simulink model "desorption_03c_sim_cl"  (R2017b)
settings: Solver=ode23s  StartTime=0.0  StopTime=tEndSimul  MaxStep=0.1  RelTol=1e-4
values from neighbouring files (symbols this model uses):
  b_motor = 1e-3    (= 0.001)    [desorption_03c_cl.m]
  c = conversion_factors()    [desorption_03c_cl.m]
  compr_water_epsilon = 0.8    [desorption_03c_cl.m]
  compr_water_flow_L_min = 10    [desorption_03c_cl.m]
  compr_water_Tin_C = Tamb_C    (= 25)    [desorption_03c_cl.m]
  fluid = nh3_v4    [desorption_03c_cl.m]
  h_liq_wall = 50    [desorption_03c_cl.m]
  h_reactor_air = h_desorp    (= 200)    [desorption_03c_cl.m]
  h_reservoir_inner_liq = 50    [desorption_03c_cl.m]
  h_reservoir_inner_vap = 10    [desorption_03c_cl.m]
  h_reservoir_outer = 10    [desorption_03c_cl.m]
  h_vap_wall = 1e4    (= 10000)    [desorption_03c_cl.m]
  h_wall_water = 200    [desorption_03c_cl.m]
  J_motor = 0.1    [desorption_03c_cl.m]
  L_min_water = L_min_water_condenser    (= 20)    [desorption_03c_cl.m]
  La_motor = 2.31e-3    (= 0.00231)    [desorption_03c_cl.m]
  motor_start_time_sec = 100 * c.min_to_sec    [desorption_03c_cl.m]
  PID_I_Tdisch = 0.01    [desorption_03c_cl.m]
  PID_P_Tdisch = 5    [desorption_03c_cl.m]
  Ra_motor = 2    [desorption_03c_cl.m]
  reservoir_L = 0.4 * Ngalettes * 46.5 * c.mm_to_m    [desorption_03c_cl.m]
  rpm_init = 0    [desorption_03c_cl.m]
  rpm_max = dVswept_rmp * 2    (= 2900)    [desorption_03c_cl.m]
  T1 = motor_start_time_sec+0    [desorption_03c_cl.m]
  Tamb_C = 25    [desorption_03c_cl.m]
  Tdesorp_source_C = Tdesorp_C    (= 25)    [desorption_03c_cl.m]
  Tdisch_ref_C = Tdisch    (= 180)    [desorption_03c_cl.m]
  Twater_in_C = 25    [desorption_03c_cl.m]
  Xend = Xinit - 0.9    (= 0.09)    [desorption_03c_cl.m]
undefined symbols (not defined in the file or in its folder): PID_D_Tdisch
libraries: thermochemical x41, simulink_extras x4, simulink x2
settings Model: Creator=ferru  LastModifiedBy=fferrucc
settings SolverCC: ZeroCrossAlgorithm=Adaptive

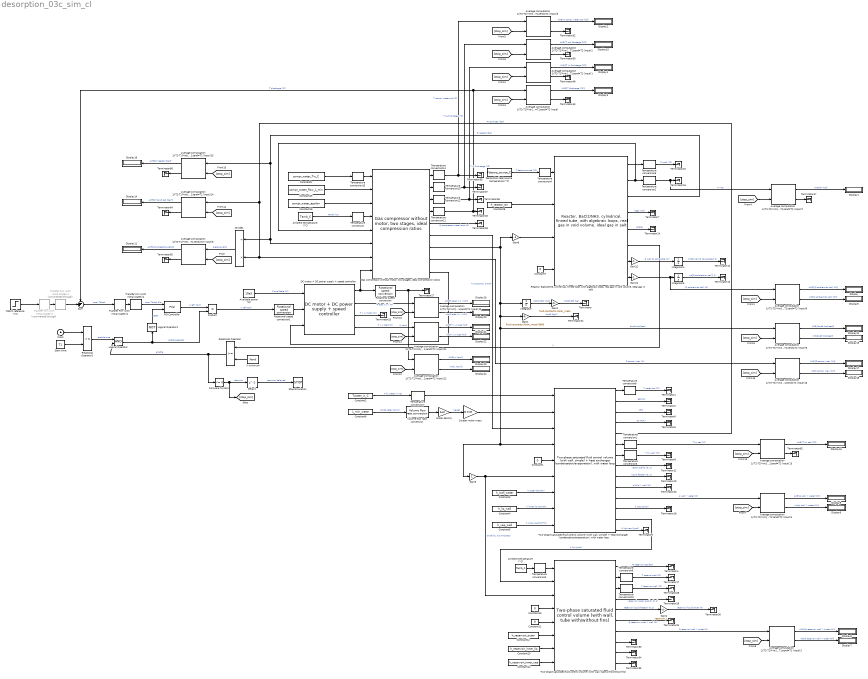
== system desorption_03c_sim_cl ==
  1/water molar mass : Gain  Gain=55.5085
  Ambient temperature (°C) : Constant  Value=Tamb_C
  "Ambient temperature (°C) " : Constant  Value=Tamb_C
  Available power (W) : Constant  Value=10e3
  Average computation 1/(T2-T1)*int{x}|t0=T1,tend=T2 (input){,1..16} (17 alike) : thermochemical/Utils/Average computation 1//(T2-T1)*int{x}|t0=T1,tend=T2 (input)  T1=T1
      settings: SourceProductName=@ Thermochemical
  Clock : Clock
  Compare To Zero : simulink/Logic and Bit Operations/Compare To Zero  relop=<=  OutDataTypeStr=boolean
  Constant{1,7,10..11} (4 alike) : Constant  Value=0
  Constant12 : Constant  Value=h_reservoir_outer
  Constant13 : Constant  Value=h_reservoir_inner_liq
  Constant14 : Constant  Value=h_reservoir_inner_vap
  Constant15 : Constant  Value=compr_water_flow_L_min
  Constant16 : Constant  Value=compr_water_epsilon
  Constant2 : Constant  Value=Twater_in_C
  Constant3 : Constant  Value=h_wall_water
  Constant4 : Constant  Value=h_liq_wall
  Constant5 : Constant  Value=h_vap_wall
  Constant6 : Constant  Value=L_min_water
  Constant8 : Constant  Value=h_reactor_air
  Constant9 : Constant  Value=compr_water_Tin_C
  DC motor + DC power supply + speed controller : thermochemical/Motors/DC motor + DC power supply +  speed controller  L=La_motor  R=Ra_motor  J=J_motor  b=b_motor  Km=Km_motor  w_init_motor=rpm_init*c.rpm_to_rad_sec  PID_P=PID_P_motor  PID_I=PID_I_motor  PID_D=PID_D_motor  V_max=Vmax_motor
      settings: SourceProductName=@ Thermochemical
  Delay1 : Delay  DelayLength=1
  Desorption heat source temperature (°C) : Constant  Value=Tdesorp_source_C
  Display{,1..24} (25 alike) : Display
  Divide1 : Product  Inputs=/*
  Gain1 : Gain  Gain=fluid.constants.Molar_mass*3600
  Gain11 : Gain  Gain=-1
  Gain12 : Gain  Gain=-1
  Gain2 : Gain  Gain=fluid.constants.Molar_mass
  Gain3 : Gain
  Gain4 : Gain  Gain=reservoir_L
  Gain6 : Gain  Gain=-1
  "Gas compressor without motor, two stages, ideal compression ratios" : thermochemical/Compression/Gas compressor without motor, two stages, ideal compression ratios  fluid=fluid  eta_IS=0.7  CL=0.03  eta_mech=0.9  dVswept_m3_h=6  dVswept_rmp=1500
      settings: SourceProductName=@ Thermochemical
  Integrator : Integrator
  Integrator4 : Integrator
  Integrator5 : Integrator
  Logical Operator : Logic  AllPortsSameDT=off  OutDataTypeStr=boolean
  Logical Operator1 : Logic  Operator=NOT  AllPortsSameDT=off  OutDataTypeStr=boolean
  PID Controller : simulink/Continuous/PID Controller  Controller=PI  TimeDomain=Continuous-time  SampleTime=-1  IntegratorMethod=Forward Euler  FilterMethod=Forward Euler  Form=Ideal  UseFilter=on  ControllerParametersSource=internal  P=PID_P_Tdisch  I=PID_I_Tdisch  D=PID_D_Tdisch  N=100  InitialConditionSource=internal  InitialConditionForIntegrator=0  InitialConditionForFilter=0  ExternalReset=level  LimitOutput=on  UpperSaturationLimit=rpm_max  LowerSaturationLimit=0  LinearizeAsGain=off  AntiWindupMode=clamping  Kb=1  TrackingMode=off  Kt=1  PParamMin=[]  PParamMax=[]  IParamMin=[]  IParamMax=[]  DParamMin=[]  DParamMax=[]  NParamMin=[]  NParamMax=[]  KbParamMin=[]  KbParamMax=[]  KtParamMin=[]  KtParamMax=[]  POutMin=[]  POutMax=[]  IOutMin=[]  IOutMax=[]  DOutMin=[]  DOutMax=[]  NOutMin=[]  NOutMax=[]  KbOutMin=[]  KbOutMax=[]  KtOutMin=[]  KtOutMax=[]  IntegratorOutMin=[]  IntegratorOutMax=[]  FilterOutMin=[]  FilterOutMax=[]  SumOutMin=[]  SumOutMax=[]  SumI1OutMin=[]  SumI1OutMax=[]  SumI2OutMin=[]  SumI2OutMax=[]  SumI3OutMin=[]  SumI3OutMax=[]  SumDOutMin=[]  SumDOutMax=[]  SaturationOutMin=[]  SaturationOutMax=[]  IntegratorContinuousStateAttributes=''  IntegratorStateMustResolveToSignalObject=off  IntegratorRTWStateStorageClass=Auto  FilterContinuousStateAttributes=''  FilterStateMustResolveToSignalObject=off  FilterRTWStateStorageClass=Auto  DifferentiatorICPrevScaledInput=0  DifferentiatorOutMin=[]  DifferentiatorOutMax=[]  InitialConditionSetting=State (most efficient)  FilterDiffOutCoefMin=[]  FilterDiffOutCoefMax=[]  SumDenOutMin=[]  SumDenOutMax=[]  SumNumOutMin=[]  SumNumOutMax=[]  ReciprocalOutMin=[]  ReciprocalOutMax=[]  DivideOutMin=[]  DivideOutMax=[]  TunerSelectOption=Transfer Function Based (PID Tuner App)
  Product : Product
  "Reactor, BaCl2/NH3, cylindrical, finned tube, with algebraic loops, real gas in void volume, ideal gas in salt" : thermochemical/Reactors/Reactor, BaCl2//NH3, with algebraic loops, real gas in void volume, ideal gas in salt/Reactor, BaCl2//NH3, cylindrical, finned tube, with algebraic loops, real gas in void volume, ideal gas in salt
      link override "Reactor, BaCl2//NH3, cylindrical, no walls, with algebraic loops, real gas in void volume, ideal gas in salt": tao_salt=param.tao_salt  rho_composite=param.rho_composite  K_cin=K_cin  fluid=fluid  Lr=param.Lr  Lr_total=param.Lr_total  Dr=param.D  Ddiff=param.Ddiff  Tr_init=param.Tr_init  X_init=param.X_init
      link override "Wall, tube with//without fins": L_m=param.Lr_total  OD_mm=OD_mm  e_mm=thickness_mm  Tinit=Treactor_wall_init  height_fin_mm=0  thickness_fin_mm=0  pitch_fin_mm=0  material_fin=Aluminum 1100  cp_fin=905.9  rho_fin=2658  lambda_fin=211.8
      settings: SourceProductName=@ Thermochemical
  Relational Operator : RelationalOperator  OutDataTypeStr=boolean  RndMeth=Simplest
  Relational Operator1 : RelationalOperator  OutDataTypeStr=boolean  RndMeth=Simplest
  Rotational speed conversion : thermochemical/Conversions/Rotational speed conversion  sel=rad/sec --> rpm
      settings: SourceProductName=@ Thermochemical
  Rotational speed conversion1 : thermochemical/Conversions/Rotational speed conversion  sel=rpm --> rad/sec
      settings: SourceProductName=@ Thermochemical
  Start time : Constant  Value=T1
  Stop Simulation : Stop
  Sum : Sum  Inputs=-+|
  Tdisch reference (°C) : Step  Time=motor_start_time_sec  Before=Tamb_C  After=Tdisch_ref_C  SampleTime=0
  Temperature conversion{,4..5,7,15} (5 alike) : thermochemical/Conversions/Temperature conversion  sel=°C --> K
      settings: SourceProductName=@ Thermochemical
  Temperature conversion{1..3,6,8..14} (11 alike) : thermochemical/Conversions/Temperature conversion  sel=K --> °C
      settings: SourceProductName=@ Thermochemical
  Terminator{,1..2,4..18,20,22,25..31,33..39,43,47..48,50,52,55,62,64,66} (43 alike) : Terminator
  Transfer Fcn (with initial states)1 : simulink_extras/Additional Linear/Transfer Fcn (with initial states)  N=[1]  D="[5  1]"  X0=0
  Transfer Fcn (with initial states)2 : simulink_extras/Additional Linear/Transfer Fcn (with initial states)  N=[1]  D="[5  1]"  X0=0
  Transfer Fcn (with initial states)3 : simulink_extras/Additional Linear/Transfer Fcn (with initial states)  Commented=through  N=[1]  D="[5  1]"  X0=Tamb_C
  Transfer Fcn (with initial states)4 : simulink_extras/Additional Linear/Transfer Fcn (with initial states)  Commented=through  N=[1]  D="[5  1]"  X0=Tamb_C
  "Two-phase saturated fluid control volume (with wall, tube with/without fins)" : thermochemical/Control volumes/Two-phase saturated fluid control volume (with wall, tube with//without fins)
      link override Two-phase saturated fluid control volume (without walls): N_init=reservoir_Ninit  T_init=reservoir_Tinit  V=reservoir_V
      link override "Wall, tube with//without fins": L_m=reservoir_L  OD_mm=reservoir_OD_mm  e_mm=reservoir_thickness_mm  material_tube=Stainless steel AISI316  cp_tube=490.8  rho_tube=8023
      settings: SourceProductName=@ Thermochemical
  "Two-phase saturated fluid control volume (with wall, simple) + heat exchanger (condensation/evaporation), with water loop" : thermochemical/Control volumes/Two-phase saturated fluid control volume (with wall, simple) + heat exchanger (condensation//evaporation), with water loop
      link override "Two-phase saturated fluid control volume (with wall, simple)/Two-phase saturated fluid control volume (without walls)": N_init=Nhx_init  T_init=Thx_init  V=Vhx
      link override "Two-phase saturated fluid control volume (with wall, simple)/Wall, simple, h as inputs": material=Stainless steel AISI316  cp=490.8  rho=8023  s=Shx_m2  e_mm=thickness_hx_mm  mass=2.2529
      settings: SourceProductName=@ Thermochemical
  Volume flow rate conversion : thermochemical/Conversions/Volume flow rate conversion  sel=L/min --> m3/sec
      settings: SourceProductName=@ Thermochemical
  Water density : Gain  Gain=1e3
  X minimum : Constant  Value=Xend
  wires:
  Integrator/1 -> Gain2/1  "int{dn/dt} (mol)"
  Temperature conversion2/1 -> "Average computation 1/(T2-T1)*int{x}|t0=T1,tend=T2 (input)7"/1, Terminator16/1  "Tr (°C)"
  Temperature conversion6/1 -> Terminator15/1  "Tr,wall (°C)"
  "Reactor, BaCl2/NH3, cylindrical, finned tube, with algebraic loops, real gas in void volume, ideal gas in salt"/4 -> Terminator7/1  "hgas void"
  "Reactor, BaCl2/NH3, cylindrical, finned tube, with algebraic loops, real gas in void volume, ideal gas in salt"/5 -> Terminator14/1  "phase"
  "Reactor, BaCl2/NH3, cylindrical, finned tube, with algebraic loops, real gas in void volume, ideal gas in salt"/2 -> "Gas compressor without motor, two stages, ideal compression ratios"/5, Temperature conversion2/1
  "Reactor, BaCl2/NH3, cylindrical, finned tube, with algebraic loops, real gas in void volume, ideal gas in salt"/6 -> Relational Operator/1  "X"
  "Reactor, BaCl2/NH3, cylindrical, finned tube, with algebraic loops, real gas in void volume, ideal gas in salt"/3 -> "Average computation 1/(T2-T1)*int{x}|t0=T1,tend=T2 (input)15"/1, Divide1/1, "Gas compressor without motor, two stages, ideal compression ratios"/6  "Pr reactor (bar)"
  "Reactor, BaCl2/NH3, cylindrical, finned tube, with algebraic loops, real gas in void volume, ideal gas in salt"/1 -> Temperature conversion6/1
  Gain11/1 -> "Average computation 1/(T2-T1)*int{x}|t0=T1,tend=T2 (input)6"/1, Integrator5/1  "Q ambient to wall (W)"
  "Reactor, BaCl2/NH3, cylindrical, finned tube, with algebraic loops, real gas in void volume, ideal gas in salt"/8 -> Gain11/1
  Integrator4/1 -> Terminator12/1  "int{Q wall to composite} (J)"
  Gain12/1 -> Integrator4/1  "Q wall to composite (W)"
  Integrator5/1 -> Terminator13/1  "int{Q ambient to wall} (J)"
  "Reactor, BaCl2/NH3, cylindrical, finned tube, with algebraic loops, real gas in void volume, ideal gas in salt"/7 -> Gain12/1
  "Two-phase saturated fluid control volume (with wall, simple) + heat exchanger (condensation/evaporation), with water loop"/10 -> Terminator20/1  "q fluid > wall (W)"
  "Two-phase saturated fluid control volume (with wall, simple) + heat exchanger (condensation/evaporation), with water loop"/9 -> Terminator10/1  "liquid fraction (0..1)"
  Water density/1 -> 1/water molar mass/1  "kg/sec"
  Temperature conversion3/1 -> Terminator8/1  "T hx,wall (°C)"
  "Two-phase saturated fluid control volume (with wall, simple) + heat exchanger (condensation/evaporation), with water loop"/11 -> "Average computation 1/(T2-T1)*int{x}|t0=T1,tend=T2 (input)4"/1  "q wall > water (W)"
  Constant2/1 -> Temperature conversion7/1  "T hx,water in (°C)"
  "Two-phase saturated fluid control volume (with wall, simple) + heat exchanger (condensation/evaporation), with water loop"/2 -> Terminator2/1  "epsilon"
  "Two-phase saturated fluid control volume (with wall, simple) + heat exchanger (condensation/evaporation), with water loop"/4 -> Terminator5/1  "UA (W/K)"
  "Two-phase saturated fluid control volume (with wall, simple) + heat exchanger (condensation/evaporation), with water loop"/12 -> Terminator18/1  "h vap (J/mol)"
  "Two-phase saturated fluid control volume (with wall, simple) + heat exchanger (condensation/evaporation), with water loop"/1 -> Temperature conversion8/1
  "Two-phase saturated fluid control volume (with wall, simple) + heat exchanger (condensation/evaporation), with water loop"/13 -> "Two-phase saturated fluid control volume (with wall, tube with/without fins)"/2  "h liq (J/mol)"
  Volume flow rate conversion/1 -> Water density/1
  "Two-phase saturated fluid control volume (with wall, simple) + heat exchanger (condensation/evaporation), with water loop"/3 -> Terminator6/1  "NTU"
  Temperature conversion8/1 -> Terminator1/1  "T water out (°C)"
  "Two-phase saturated fluid control volume (with wall, simple) + heat exchanger (condensation/evaporation), with water loop"/6 -> Temperature conversion1/1
  "Two-phase saturated fluid control volume (with wall, simple) + heat exchanger (condensation/evaporation), with water loop"/14 -> Terminator9/1  "h liq+vap (J/mol)"
  Constant4/1 -> "Two-phase saturated fluid control volume (with wall, simple) + heat exchanger (condensation/evaporation), with water loop"/8  "h inner liq (W/m²/K)"
  Constant5/1 -> "Two-phase saturated fluid control volume (with wall, simple) + heat exchanger (condensation/evaporation), with water loop"/9  "h inner vap(W/m²/K)"
  "Two-phase saturated fluid control volume (with wall, simple) + heat exchanger (condensation/evaporation), with water loop"/7 -> Temperature conversion3/1
  Constant3/1 -> "Two-phase saturated fluid control volume (with wall, simple) + heat exchanger (condensation/evaporation), with water loop"/7  "h outer (W/m²/K)"
  Temperature conversion1/1 -> "Average computation 1/(T2-T1)*int{x}|t0=T1,tend=T2 (input)13"/1  "T hx,sat (°C)"
  "Two-phase saturated fluid control volume (with wall, simple) + heat exchanger (condensation/evaporation), with water loop"/8 -> Terminator11/1  "vapor quality (0..1)"
  Gain3/1 -> "Two-phase saturated fluid control volume (with wall, tube with/without fins)"/3, "Two-phase saturated fluid control volume (with wall, simple) + heat exchanger (condensation/evaporation), with water loop"/6  "dn/dt liq, out (mol/sec)"
  Temperature conversion7/1 -> "Two-phase saturated fluid control volume (with wall, simple) + heat exchanger (condensation/evaporation), with water loop"/1
  "Gas compressor without motor, two stages, ideal compression ratios"/8 -> "Average computation 1/(T2-T1)*int{x}|t0=T1,tend=T2 (input)16"/1  "P compr. irrev (W)"
  Rotational speed conversion1/1 -> DC motor + DC power supply + speed controller/2
  DC motor + DC power supply + speed controller/3 -> Terminator25/1  "T x w motor (W)"
  Temperature conversion11/1 -> Sum/1, "Average computation 1/(T2-T1)*int{x}|t0=T1,tend=T2 (input)"/1, Terminator26/1  "T discharge (°C)"
  Rotational speed conversion/1 -> "Average computation 1/(T2-T1)*int{x}|t0=T1,tend=T2 (input)12"/1, Terminator27/1  "w (rpm)"
  Temperature conversion/1 -> "Gas compressor without motor, two stages, ideal compression ratios"/4
  "Gas compressor without motor, two stages, ideal compression ratios"/4 -> Temperature conversion11/1
  "Gas compressor without motor, two stages, ideal compression ratios"/9 -> DC motor + DC power supply + speed controller/3
  Ambient temperature (°C)/1 -> Temperature conversion/1  "Tamb (°C)"
  Available power (W)/1 -> DC motor + DC power supply + speed controller/1  "P available (W)"
  DC motor + DC power supply + speed controller/1 -> "Gas compressor without motor, two stages, ideal compression ratios"/8, Rotational speed conversion/1
  Product/1 -> Rotational speed conversion1/1  "w ref (rpm)"
  "Gas compressor without motor, two stages, ideal compression ratios"/7 -> Gain6/1, "Average computation 1/(T2-T1)*int{x}|t0=T1,tend=T2 (input)9"/1, Gain3/1, "Two-phase saturated fluid control volume (with wall, simple) + heat exchanger (condensation/evaporation), with water loop"/4, Gain1/1, Integrator/1  "dn/dt (mol/sec)"
  Constant7/1 -> "Reactor, BaCl2/NH3, cylindrical, finned tube, with algebraic loops, real gas in void volume, ideal gas in salt"/4
  Gain6/1 -> "Reactor, BaCl2/NH3, cylindrical, finned tube, with algebraic loops, real gas in void volume, ideal gas in salt"/3
  "Gas compressor without motor, two stages, ideal compression ratios"/6 -> "Two-phase saturated fluid control volume (with wall, simple) + heat exchanger (condensation/evaporation), with water loop"/3  "h out compr. (J/mol)"
  Constant1/1 -> "Two-phase saturated fluid control volume (with wall, simple) + heat exchanger (condensation/evaporation), with water loop"/5
  Constant6/1 -> Volume flow rate conversion/1  "dV/dt water (L/min)"
  1/water molar mass/1 -> "Two-phase saturated fluid control volume (with wall, simple) + heat exchanger (condensation/evaporation), with water loop"/2
  Desorption heat source temperature (°C)/1 -> Temperature conversion4/1  "T desorp,source (°C)"
  Temperature conversion4/1 -> "Reactor, BaCl2/NH3, cylindrical, finned tube, with algebraic loops, real gas in void volume, ideal gas in salt"/1
  Constant8/1 -> "Reactor, BaCl2/NH3, cylindrical, finned tube, with algebraic loops, real gas in void volume, ideal gas in salt"/2
  Gain1/1 -> Terminator22/1  "dn/dt (kg/h)"
  Gain2/1 -> Terminator/1  "int{dn/dt} (kg)"
  "Ambient temperature (°C) "/1 -> Temperature conversion5/1
  Temperature conversion5/1 -> "Two-phase saturated fluid control volume (with wall, tube with/without fins)"/1
  Constant10/1 -> "Two-phase saturated fluid control volume (with wall, tube with/without fins)"/4
  Constant11/1 -> "Two-phase saturated fluid control volume (with wall, tube with/without fins)"/5
  Constant12/1 -> "Two-phase saturated fluid control volume (with wall, tube with/without fins)"/6
  Constant13/1 -> "Two-phase saturated fluid control volume (with wall, tube with/without fins)"/7
  Constant14/1 -> "Two-phase saturated fluid control volume (with wall, tube with/without fins)"/8
  "Two-phase saturated fluid control volume (with wall, tube with/without fins)"/1 -> Terminator4/1  "Pr reservoir sat (bar)"
  Temperature conversion9/1 -> Terminator17/1  "T reservoir sat (°C)"
  "Two-phase saturated fluid control volume (with wall, tube with/without fins)"/3 -> Temperature conversion10/1
  "Two-phase saturated fluid control volume (with wall, tube with/without fins)"/5 -> Gain4/1  "reservoir liquid fraction (0..1)"
  "Two-phase saturated fluid control volume (with wall, tube with/without fins)"/6 -> Terminator31/1  "Q reservoir inner > wall (W)"
  "Two-phase saturated fluid control volume (with wall, tube with/without fins)"/7 -> "Average computation 1/(T2-T1)*int{x}|t0=T1,tend=T2 (input)3"/1  "Q reservoir wall > outer (W)"
  "Two-phase saturated fluid control volume (with wall, tube with/without fins)"/8 -> Terminator33/1
  "Two-phase saturated fluid control volume (with wall, tube with/without fins)"/9 -> Terminator34/1
  "Two-phase saturated fluid control volume (with wall, tube with/without fins)"/10 -> Terminator35/1
  "Two-phase saturated fluid control volume (with wall, tube with/without fins)"/2 -> Temperature conversion9/1
  Temperature conversion10/1 -> Terminator28/1  "T reservoir wall (°C)"
  "Two-phase saturated fluid control volume (with wall, tube with/without fins)"/4 -> Terminator29/1  "reservoir vapor quality (0..1)"
  Gain4/1 -> Terminator30/1  "reservoir liquid level (m)"
  X minimum/1 -> Relational Operator/2
  Relational Operator/1 -> Logical Operator/2, Compare To Zero/1  "enable"
  "Two-phase saturated fluid control volume (with wall, simple) + heat exchanger (condensation/evaporation), with water loop"/5 -> "Average computation 1/(T2-T1)*int{x}|t0=T1,tend=T2 (input)14"/1, "Gas compressor without motor, two stages, ideal compression ratios"/7, Divide1/2  "Pr cond sat. (bar)"
  Temperature conversion12/1 -> "Average computation 1/(T2-T1)*int{x}|t0=T1,tend=T2 (input)1"/1, Terminator36/1  "T in 2nd stage (°C)"
  "Gas compressor without motor, two stages, ideal compression ratios"/3 -> Temperature conversion12/1
  Temperature conversion13/1 -> "Average computation 1/(T2-T1)*int{x}|t0=T1,tend=T2 (input)2"/1, Terminator37/1  "T out 1st stage (°C)"
  Temperature conversion14/1 -> "Average computation 1/(T2-T1)*int{x}|t0=T1,tend=T2 (input)5"/1, Terminator38/1  "T compr. water out (°C)"
  "Gas compressor without motor, two stages, ideal compression ratios"/1 -> Temperature conversion14/1
  "Gas compressor without motor, two stages, ideal compression ratios"/2 -> Temperature conversion13/1
  "Gas compressor without motor, two stages, ideal compression ratios"/5 -> Terminator39/1  "Q compressor water loop (W)"
  Temperature conversion15/1 -> "Gas compressor without motor, two stages, ideal compression ratios"/1
  Constant9/1 -> Temperature conversion15/1
  Constant15/1 -> "Gas compressor without motor, two stages, ideal compression ratios"/2
  Constant16/1 -> "Gas compressor without motor, two stages, ideal compression ratios"/3
  "Average computation 1/(T2-T1)*int{x}|t0=T1,tend=T2 (input)7"/2 -> Terminator47/1
  [stop_sim] -> "Average computation 1/(T2-T1)*int{x}|t0=T1,tend=T2 (input)7"/2
  "Average computation 1/(T2-T1)*int{x}|t0=T1,tend=T2 (input)7"/1 -> Display4/1  "AVG{Tr (°C)}"
  [stop_sim] -> "Average computation 1/(T2-T1)*int{x}|t0=T1,tend=T2 (input)6"/2
  "Average computation 1/(T2-T1)*int{x}|t0=T1,tend=T2 (input)6"/1 -> Display/1  "AVG{Q ambient to wall (W)}"
  "Average computation 1/(T2-T1)*int{x}|t0=T1,tend=T2 (input)6"/2 -> Display5/1  "int{Q ambient to wall (W)}"
  [stop_sim] -> "Average computation 1/(T2-T1)*int{x}|t0=T1,tend=T2 (input)4"/2
  "Average computation 1/(T2-T1)*int{x}|t0=T1,tend=T2 (input)4"/2 -> Display6/1  "int{q wall > water (W)}"
  "Average computation 1/(T2-T1)*int{x}|t0=T1,tend=T2 (input)4"/1 -> Display9/1  "AVG{q wall > water (W)}"
  "Average computation 1/(T2-T1)*int{x}|t0=T1,tend=T2 (input)3"/1 -> Display8/1  "AVG{Q reservoir wall > outer (W)}"
  "Average computation 1/(T2-T1)*int{x}|t0=T1,tend=T2 (input)3"/2 -> Display7/1  "int{Q reservoir wall > outer (W)}"
  [stop_sim] -> "Average computation 1/(T2-T1)*int{x}|t0=T1,tend=T2 (input)3"/2
  "Average computation 1/(T2-T1)*int{x}|t0=T1,tend=T2 (input)"/2 -> Terminator43/1
  "Average computation 1/(T2-T1)*int{x}|t0=T1,tend=T2 (input)"/1 -> Display3/1  "AVG{T discharge (°C)}"
  [stop_sim] -> "Average computation 1/(T2-T1)*int{x}|t0=T1,tend=T2 (input)"/2
  [stop_sim] -> "Average computation 1/(T2-T1)*int{x}|t0=T1,tend=T2 (input)1"/2
  "Average computation 1/(T2-T1)*int{x}|t0=T1,tend=T2 (input)1"/1 -> Display1/1  "AVG{T in 2nd stage (°C)}"
  "Average computation 1/(T2-T1)*int{x}|t0=T1,tend=T2 (input)1"/2 -> Terminator48/1
  "Average computation 1/(T2-T1)*int{x}|t0=T1,tend=T2 (input)5"/2 -> Terminator52/1
  "Average computation 1/(T2-T1)*int{x}|t0=T1,tend=T2 (input)5"/1 -> Display2/1  "AVG{T compr. water out (°C)}"
  [stop_sim] -> "Average computation 1/(T2-T1)*int{x}|t0=T1,tend=T2 (input)5"/2
  [stop_sim] -> "Average computation 1/(T2-T1)*int{x}|t0=T1,tend=T2 (input)2"/2
  "Average computation 1/(T2-T1)*int{x}|t0=T1,tend=T2 (input)2"/1 -> Display10/1  "AVG{T out 1st stage (°C)}"
  "Average computation 1/(T2-T1)*int{x}|t0=T1,tend=T2 (input)2"/2 -> Terminator50/1
  [stop_sim] -> "Average computation 1/(T2-T1)*int{x}|t0=T1,tend=T2 (input)8"/2
  Divide1/1 -> "Average computation 1/(T2-T1)*int{x}|t0=T1,tend=T2 (input)8"/1  "pressure ratio"
  "Average computation 1/(T2-T1)*int{x}|t0=T1,tend=T2 (input)8"/2 -> Terminator55/1
  "Average computation 1/(T2-T1)*int{x}|t0=T1,tend=T2 (input)8"/1 -> Display11/1  "AVG{compresssion_ratio}"
  Delay1/1 -> Stop Simulation/1  "stop sim delayed"
  Compare To Zero/1 -> [stop_sim], Delay1/1  "stop sim"
  "Average computation 1/(T2-T1)*int{x}|t0=T1,tend=T2 (input)9"/2 -> Display13/1  "int{dn/dt (mol/sec)}"
  [stop_sim] -> "Average computation 1/(T2-T1)*int{x}|t0=T1,tend=T2 (input)9"/2
  "Average computation 1/(T2-T1)*int{x}|t0=T1,tend=T2 (input)9"/1 -> Display12/1  "AVG{dn/dt (mol/sec)}"
  "Average computation 1/(T2-T1)*int{x}|t0=T1,tend=T2 (input)11"/2 -> Display22/1  "int{T x w load (W)}"
  DC motor + DC power supply + speed controller/2 -> "Average computation 1/(T2-T1)*int{x}|t0=T1,tend=T2 (input)10"/1  "P elec: U x I (W)"
  "Average computation 1/(T2-T1)*int{x}|t0=T1,tend=T2 (input)11"/1 -> Display21/1  "AVG{T x w load (W)}"
  [stop_sim] -> "Average computation 1/(T2-T1)*int{x}|t0=T1,tend=T2 (input)10"/2
  "Average computation 1/(T2-T1)*int{x}|t0=T1,tend=T2 (input)10"/2 -> Display20/1  "int{P elec: U x I (W)}"
  DC motor + DC power supply + speed controller/4 -> "Average computation 1/(T2-T1)*int{x}|t0=T1,tend=T2 (input)11"/1  "T x w load (W)"
  [stop_sim] -> "Average computation 1/(T2-T1)*int{x}|t0=T1,tend=T2 (input)11"/2
  "Average computation 1/(T2-T1)*int{x}|t0=T1,tend=T2 (input)10"/1 -> Display19/1  "AVG{P elec: U x I (W)}"
  Tdisch reference (°C)/1 -> Transfer Fcn (with initial states)3/1
  Start time/1 -> Relational Operator1/2
  Logical Operator/1 -> Product/2, Logical Operator1/1  "enable general"
  Relational Operator1/1 -> Logical Operator/1  "enable time"
  PID Controller/1 -> Product/1  "w ref* (rpm)"
  Clock/1 -> Relational Operator1/1
  Transfer Fcn (with initial states)1/1 -> Transfer Fcn (with initial states)2/1
  Sum/1 -> Transfer Fcn (with initial states)1/1  "error Tdisch"
  Logical Operator1/1 -> PID Controller/2  "reset"
  Transfer Fcn (with initial states)2/1 -> PID Controller/1  "error Tdisch filtr"
  [stop_sim] -> "Average computation 1/(T2-T1)*int{x}|t0=T1,tend=T2 (input)12"/2
  "Average computation 1/(T2-T1)*int{x}|t0=T1,tend=T2 (input)12"/1 -> Display23/1  "AVG{w (rpm)}"
  "Average computation 1/(T2-T1)*int{x}|t0=T1,tend=T2 (input)12"/2 -> Display24/1  "int{w (rpm)}"
  "Average computation 1/(T2-T1)*int{x}|t0=T1,tend=T2 (input)13"/1 -> Display15/1  "AVG{T hx,sat (°C)}"
  "Average computation 1/(T2-T1)*int{x}|t0=T1,tend=T2 (input)13"/2 -> Terminator62/1
  [stop_sim] -> "Average computation 1/(T2-T1)*int{x}|t0=T1,tend=T2 (input)13"/2
  "Average computation 1/(T2-T1)*int{x}|t0=T1,tend=T2 (input)14"/1 -> Display14/1  "AVG{Pr cond sat. (bar)}"
  "Average computation 1/(T2-T1)*int{x}|t0=T1,tend=T2 (input)14"/2 -> Terminator64/1
  [stop_sim] -> "Average computation 1/(T2-T1)*int{x}|t0=T1,tend=T2 (input)14"/2
  [stop_sim] -> "Average computation 1/(T2-T1)*int{x}|t0=T1,tend=T2 (input)15"/2
  "Average computation 1/(T2-T1)*int{x}|t0=T1,tend=T2 (input)15"/2 -> Terminator66/1
  "Average computation 1/(T2-T1)*int{x}|t0=T1,tend=T2 (input)15"/1 -> Display16/1  "AVG{Pr reactor (bar)}"
  Transfer Fcn (with initial states)3/1 -> Transfer Fcn (with initial states)4/1
  Transfer Fcn (with initial states)4/1 -> Sum/2
  "Average computation 1/(T2-T1)*int{x}|t0=T1,tend=T2 (input)16"/1 -> Display17/1  "AVG{P compr. irrev (W)}"
  [stop_sim] -> "Average computation 1/(T2-T1)*int{x}|t0=T1,tend=T2 (input)16"/2
  "Average computation 1/(T2-T1)*int{x}|t0=T1,tend=T2 (input)16"/2 -> Display18/1  "int{P compr. irrev (W)}"
